simulink model "PedalMapping"  (R2020a)
settings: Solver=FixedStepDiscrete  StartTime=0.0  StopTime=10.0  FixedStep=ModelSimTime  RelTol=1e-3  EnableMultiTasking=on
PostLoadFcn:
  | , if any(exist('dsrtsu_mdlpostloadfcn', 'file') == [2, 3, 6]), try dsrtsu_mdlpostloadfcn('Execute', bdroot); catch fprintf('Error in PostLoadFcn (dsrtsu_mdlpostloadfcn) for model "%s":\n %s\n', bdroot, lasterr); end, end,
InitFcn:
  | , if any(exist('rtifpga_mdlclblib', 'file') ~= 0), rtifpga_mdlclblib('Init', bdroot); end,
settings Model: DSRTSU_INTERNAL_RTI_VER=560  DSRTSU_INTERNAL_RTI_TYPE=rti1401  RTICANMMDATA=struct('GeneralSetupData',struct('modelroot','C:\Users\harjo\Git\MACFormulaGit\MicroAutobox\rings\Vehicle_Dynamics_Ring','generalsettings',struct('filesettings',struct('destfolder',struct('Name','RTICANMM_FILES','Check',1),'buildfolder',struct('Name','.','Check',1),'AbsDestfolder',struct('Name','C:\Users\harjo\Git\MACFormulaGit\MicroAutobox\rings\Vehicle_Dynamics_Ring\RTICANMM_FILES'),'AbsBuildfolder',struct('Name','C:\Users\harjo\Git\MACFormulaGit\MicroAutobox\rings\Vehicle_Dynamics_Ring'))),'options',struct('addpaths',1,'rmpaths',1,'addtrcexclusion',true,'cannavigator',struct('checkmonitoring',0),'show_usrtrc',0,'use_usrtrc',0),'advanced',struct('options',ones(1,100)),'MPSetup',{{}},'RTI',struct('Type','RTI1401','Ver','7.14','Date','02-May-2020'),'modelname','PedalMapping','block','PedalMapping'))  DSRTSU_INTERNAL_RTIFPGA=160  Creator=Harjot  LastModifiedBy=Harjot
settings DebuggingCC: SFUnexpectedBacktrackingDiag=warning  SFNoUnconditionalDefaultTransitionDiag=warning  SFExecutionAtInitializationDiag=none  ArithmeticOperatorsInVariantConditions=warning
settings HardwareCC: ProdBitPerPointer=32  ProdBitPerSizeT=32  ProdBitPerPtrDiffT=32  ProdLargestAtomicInteger=Integer  ProdEndianess=BigEndian  ProdWordSize=32  ProdHWDeviceType=Custom Processor->Custom  TargetIntDivRoundTo=Zero  TargetEndianess=BigEndian  TargetHWDeviceType=Custom Processor->Custom
settings SFSimCC: SimUseLocalCustomCode=off  MATLABDynamicMemAlloc=off  CustomCodeUndefinedFunction=UseInterfaceOnly
settings RTWCC: Description=dSPACE DS1401 Hardware Platform  SystemTargetFile=rti1401.tlc  MakeCommand=make_rti  TemplateMakefile=rti1401.tmf  RTWUseLocalCustomCode=off
settings CodeAppCC: StateflowObjectComments=on
settings STFCustomTargetCC: ParMdlRefBuildCompliant=on  MatFileLogging=on  SystemTargetFile=rti1401.tlc
settings GRTTargetCC: TargetLangStandard=C89/C90 (ANSI)  CompOptLevelCompliant=off  ConcurrentExecutionCompliant=off  CombineOutputUpdateFcns=off  CPPClassGenCompliant=off  UseToolchainInfoCompliant=off
settings ConfigComp: CovMetricSettings=dw  CovHtmlReporting=on  CovSaveCumulativeToWorkspaceVar=on  CovSaveSingleToWorkspaceVar=on  CovExternalEMLEnable=off

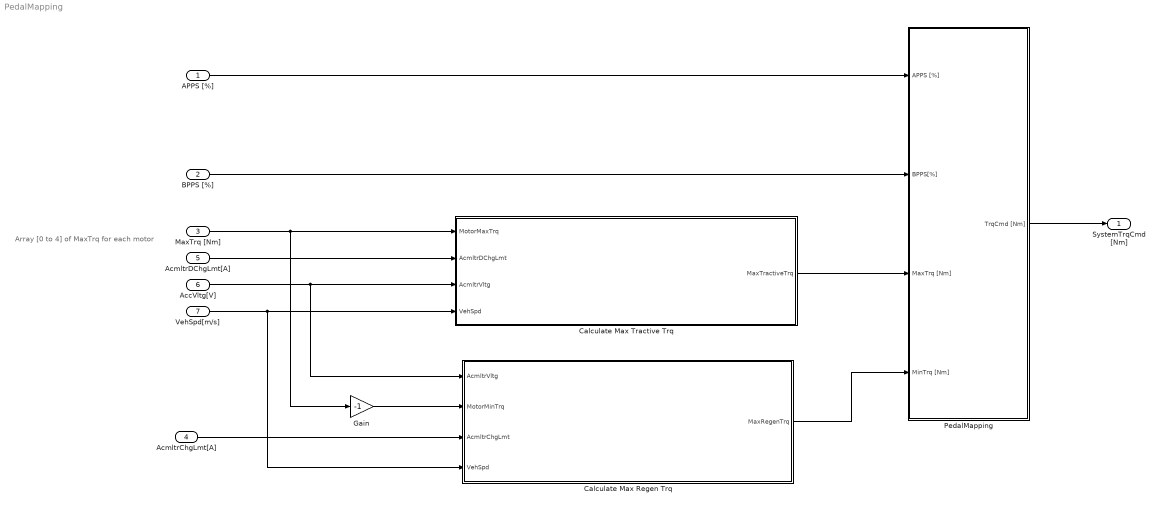
== system PedalMapping ==
  note: Array [0 to 4] of MaxTrq for each motor
  APPS [%] : Inport
  BPPS [%] : Inport  Port=2  OutDataTypeStr=double
  MaxTrq [Nm] : Inport  Port=3  PortDimensions=4
  AcmltrChgLmt[A] : Inport  Port=4  OutDataTypeStr=double
  AcmltrDChgLmt[A] : Inport  Port=5  OutDataTypeStr=double
  AccVltg[V] : Inport  Port=6
  VehSpd[m/s] : Inport  Port=7
  Calculate Max Regen Trq : Subsystem
  Calculate Max Tractive Trq : Subsystem
  Gain : Gain  Gain=-1
  PedalMapping : Subsystem
  SystemTrqCmd [Nm] : Outport  VectorParamsAs1DForOutWhenUnconnected=off
  wires:
  MaxTrq [Nm]/1 -> Gain/1, Calculate Max Tractive Trq/1(MotorMaxTrq)
  Gain/1 -> Calculate Max Regen Trq/2("MotorMinTrq ")
  AcmltrChgLmt[A]/1 -> Calculate Max Regen Trq/3(AcmltrChgLmt)
  VehSpd[m/s]/1 -> Calculate Max Regen Trq/4(VehSpd), Calculate Max Tractive Trq/4(VehSpd)
  AcmltrDChgLmt[A]/1 -> Calculate Max Tractive Trq/2(AcmltrDChgLmt)
  PedalMapping/1(TrqCmd [Nm]) -> SystemTrqCmd [Nm]/1
  AccVltg[V]/1 -> Calculate Max Regen Trq/1(AcmltrVltg), Calculate Max Tractive Trq/3(AcmltrVltg)
  APPS [%]/1 -> PedalMapping/1(APPS [%])
  BPPS [%]/1 -> PedalMapping/2(BPPS[%])
  Calculate Max Tractive Trq/1(MaxTractiveTrq) -> PedalMapping/3(MaxTrq [Nm])
  Calculate Max Regen Trq/1(MaxRegenTrq) -> PedalMapping/4(MinTrq [Nm])

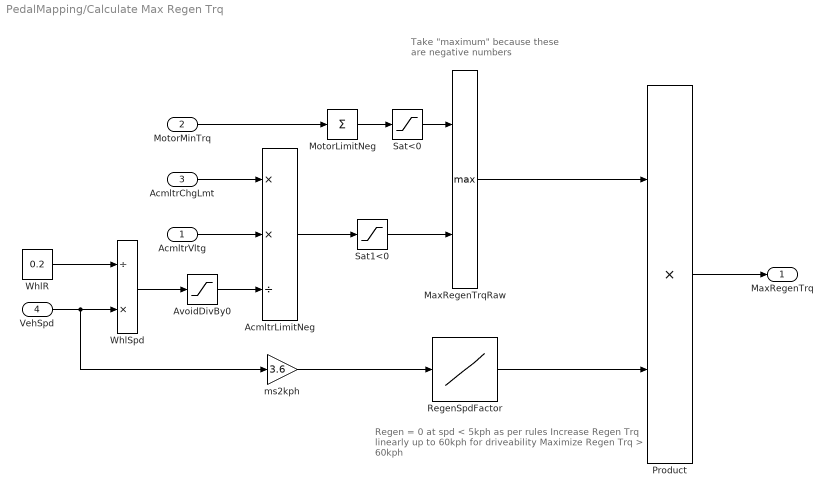
== system PedalMapping/Calculate Max Regen Trq ==
  note: Regen = 0 at spd < 5kph as per rules
      | Increase Regen Trq linearly up to 60kph for driveability
      | Maximize Regen Trq > 60kph
  note: Take "maximum" because these are negative numbers
  AcmltrVltg : Inport
  "MotorMinTrq " : Inport  Port=2
  AcmltrChgLmt : Inport  Port=3
  VehSpd : Inport  Port=4
  AcmltrLimitNeg : Product  Inputs=**/  OutDataTypeStr=double
  AvoidDivBy0 : Saturate  UpperLimit=inf  LowerLimit=1E-7
  MaxRegenTrqRaw : MinMax  Function=max  Inputs=2
  MotorLimitNeg : Sum  Inputs=+
  Product : Product
  RegenSpdFactor : Lookup_n-D  NumberOfTableDimensions=1  BreakpointsForDimension1=[0 5 60 999]  Table=[0 0 1 1]  InternalRulePriority=Speed  RndMeth=Simplest  InputSameDT=on
  Sat1<0 : Saturate  UpperLimit=0  LowerLimit=-100000
  Sat<0 : Saturate  UpperLimit=0  LowerLimit=-inf
  WhlR : Constant  Value=0.2
  WhlSpd : Product  Inputs=/*
  ms2kph : Gain  Gain=3.6
  MaxRegenTrq : Outport  VectorParamsAs1DForOutWhenUnconnected=off
  wires:
  Sat1<0/1 -> MaxRegenTrqRaw/2
  Sat<0/1 -> MaxRegenTrqRaw/1
  AvoidDivBy0/1 -> AcmltrLimitNeg/3
  WhlR/1 -> WhlSpd/1
  WhlSpd/1 -> AvoidDivBy0/1
  MotorLimitNeg/1 -> Sat<0/1
  AcmltrChgLmt/1 -> AcmltrLimitNeg/1
  VehSpd/1 -> WhlSpd/2, ms2kph/1
  AcmltrVltg/1 -> AcmltrLimitNeg/2
  Product/1 -> MaxRegenTrq/1
  ms2kph/1 -> RegenSpdFactor/1
  AcmltrLimitNeg/1 -> Sat1<0/1
  RegenSpdFactor/1 -> Product/2
  MaxRegenTrqRaw/1 -> Product/1
  "MotorMinTrq "/1 -> MotorLimitNeg/1

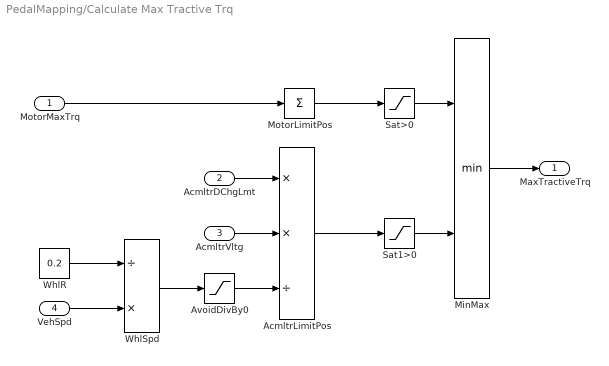
== system PedalMapping/Calculate Max Tractive Trq ==
  MotorMaxTrq : Inport
  AcmltrDChgLmt : Inport  Port=2
  AcmltrVltg : Inport  Port=3
  VehSpd : Inport  Port=4
  AcmltrLimitPos : Product  Inputs=**/  OutDataTypeStr=double
  AvoidDivBy0 : Saturate  UpperLimit=inf  LowerLimit=1E-7
  MinMax : MinMax  Inputs=2
  MotorLimitPos : Sum  Inputs=+
  Sat1>0 : Saturate  UpperLimit=100000  LowerLimit=0
  Sat>0 : Saturate  UpperLimit=inf  LowerLimit=0
  WhlR : Constant  Value=0.2
  WhlSpd : Product  Inputs=/*
  MaxTractiveTrq : Outport  VectorParamsAs1DForOutWhenUnconnected=off
  wires:
  AcmltrLimitPos/1 -> Sat1>0/1
  AvoidDivBy0/1 -> AcmltrLimitPos/3
  WhlR/1 -> WhlSpd/1
  WhlSpd/1 -> AvoidDivBy0/1
  VehSpd/1 -> WhlSpd/2
  Sat1>0/1 -> MinMax/2
  Sat>0/1 -> MinMax/1
  MotorLimitPos/1 -> Sat>0/1
  AcmltrVltg/1 -> AcmltrLimitPos/2
  AcmltrDChgLmt/1 -> AcmltrLimitPos/1
  MotorMaxTrq/1 -> MotorLimitPos/1
  MinMax/1 -> MaxTractiveTrq/1

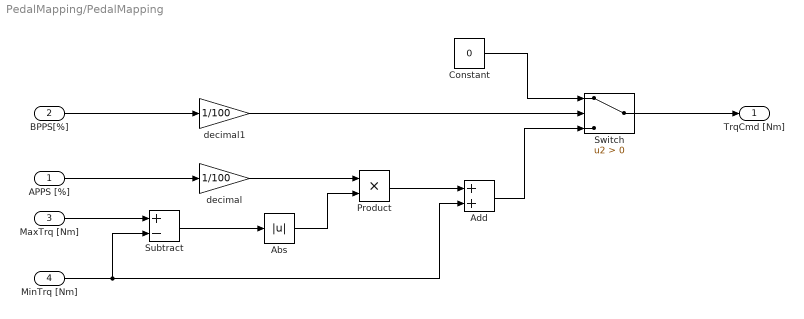
== system PedalMapping/PedalMapping ==
  APPS [%] : Inport
  BPPS[%] : Inport  Port=2
  MaxTrq [Nm] : Inport  Port=3
  MinTrq [Nm] : Inport  Port=4
  Abs : Abs
  Add : Sum
  Constant : Constant  Value=0
  Product : Product
  Subtract : Sum  Inputs=+-
  Switch : Switch  Criteria=u2 > Threshold
  decimal : Gain  Gain=1/100
  decimal1 : Gain  Gain=1/100
  TrqCmd [Nm] : Outport  VectorParamsAs1DForOutWhenUnconnected=off
  wires:
  decimal/1 -> Product/1
  Abs/1 -> Product/2
  APPS [%]/1 -> decimal/1
  MaxTrq [Nm]/1 -> Subtract/1
  Subtract/1 -> Abs/1
  MinTrq [Nm]/1 -> Add/2, Subtract/2
  BPPS[%]/1 -> decimal1/1
  Switch/1 -> TrqCmd [Nm]/1
  Add/1 -> Switch/3
  Constant/1 -> Switch/1
  Product/1 -> Add/1
  decimal1/1 -> Switch/2
